simulink library "pbbs_new"  (Simulink 8.1)
settings: Solver=ode1  StartTime=0.0  StopTime=Inf  FixedStep=0.001  RelTol=1e-3
PostLoadFcn:
  | , if any(exist('dsrtsu_mdlpostloadfcn', 'file') == [2, 3, 6]), try dsrtsu_mdlpostloadfcn('Execute', bdroot); catch fprintf('Error in PostLoadFcn (dsrtsu_mdlpostloadfcn) for model "%s":\n %s\n', bdroot, lasterr); end, end,
undefined symbols (not defined in the file or in its folder): KJUD_DecelTGapBraking_s, KJUD_SDFDelay_s, ZERO_FLOAT
libraries: ebdc x1, frdc x1, tbdc x1
settings Model: DSRTSU_INTERNAL_RTI_VER=450  DSRTSU_INTERNAL_RTI_TYPE=rti1401  RTICANMMDATA=struct('GeneralSetupData',struct('modelroot','D:\ELN150201_TAIWAN\trunk\AdasDragon\software\sw_development\arch\app\jud','generalsettings',struct('filesettings',struct('destfolder',struct('Name','RTICANMM_FILES','Check',1),'buildfolder',struct('Name','.','Check',1),'AbsDestfolder',struct('Name','D:\ELN150201_TAIWAN\trunk\AdasDragon\software\sw_development\arch\app\jud\RTICANMM_FILES'),'AbsBuildfolder',struct('Name','D:\ELN150201_TAIWAN\trunk\AdasDragon\software\sw_development\arch\app\jud'))),'options',struct('addpaths',1,'rmpaths',1,'addtrcexclusion',logical(1),'cannavigator',struct('checkmonitoring',0),'show_usrtrc',0,'use_usrtrc',0),'advanced',struct('options',[1 1 1 1 1 1 1 1 1 1 1 1 1 1 1 1 1 1 1 1 1 1 1 1 1 1 1 1 1 1 1 1 1 1 1 1 1 1 1 1 1 1 1 1 1 1 1 1 1 1 1 1 1 1 1 1 1 1 1 1 1 1 1 1 1 1 1 1 1 1 1 1 1 1 1 1 1 1 1 1 1 1 1 1 1 1 1 1 1 1 1 1 1 1 1 1 1 1 1 1]),'MPSetup',{{}},'modelname','pbbs_new','block','pbbs_new'))  DSRTSU_INTERNAL_RTIFPGA=40  Creator=tescamilla  LastModifiedBy=AT015555

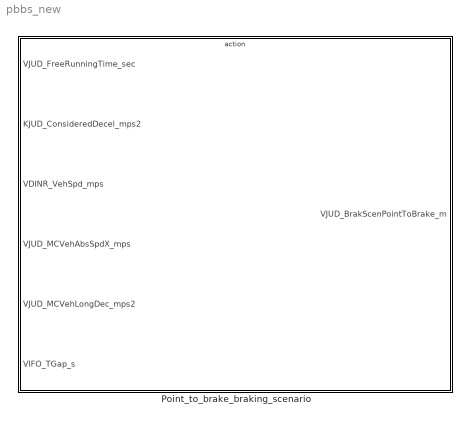
== system pbbs_new ==
  Point_to_brake_braking_scenario : Subsystem

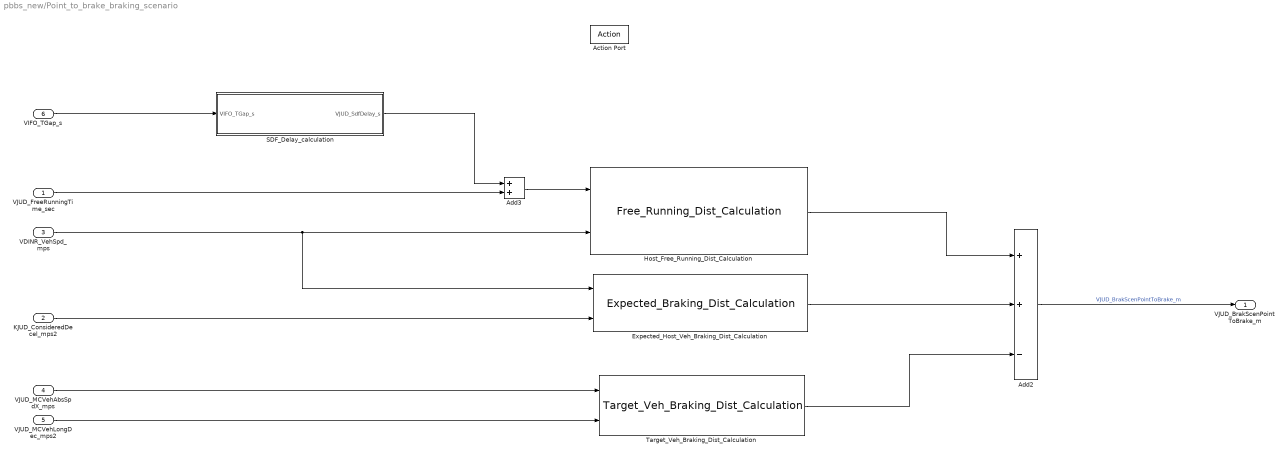
== system pbbs_new/Point_to_brake_braking_scenario ==
  VJUD_FreeRunningTime_sec : Inport
  KJUD_ConsideredDecel_mps2 : Inport  Port=2
  VDINR_VehSpd_mps : Inport  Port=3
  VJUD_MCVehAbsSpdX_mps : Inport  Port=4
  VJUD_MCVehLongDec_mps2 : Inport  Port=5
  VIFO_TGap_s : Inport  Port=6
  Action Port : ActionPort
  Add2 : Sum  Inputs=++-
  Add3 : Sum
  Expected_Host_Veh_Braking_Dist_Calculation : ebdc/Expected_Braking_Dist_Calculation
  Host_Free_Running_Dist_Calculation : frdc/Free_Running_Dist_Calculation
  SDF_Delay_calculation : Subsystem
  Target_Veh_Braking_Dist_Calculation : tbdc/Target_Veh_Braking_Dist_Calculation
  VJUD_BrakScenPointToBrake_m : Outport
  wires:
  KJUD_ConsideredDecel_mps2/1 -> Expected_Host_Veh_Braking_Dist_Calculation/2
  VJUD_FreeRunningTime_sec/1 -> Add3/2
  VDINR_VehSpd_mps/1 -> Expected_Host_Veh_Braking_Dist_Calculation/1, Host_Free_Running_Dist_Calculation/2
  VJUD_MCVehLongDec_mps2/1 -> Target_Veh_Braking_Dist_Calculation/2
  VJUD_MCVehAbsSpdX_mps/1 -> Target_Veh_Braking_Dist_Calculation/1
  Expected_Host_Veh_Braking_Dist_Calculation/1 -> Add2/2
  Host_Free_Running_Dist_Calculation/1 -> Add2/1
  Target_Veh_Braking_Dist_Calculation/1 -> Add2/3
  Add2/1 -> VJUD_BrakScenPointToBrake_m/1  "VJUD_BrakScenPointToBrake_m"
  Add3/1 -> Host_Free_Running_Dist_Calculation/1
  VIFO_TGap_s/1 -> SDF_Delay_calculation/1(VIFO_TGap_s)
  SDF_Delay_calculation/1(VJUD_SdfDelay_s) -> Add3/1

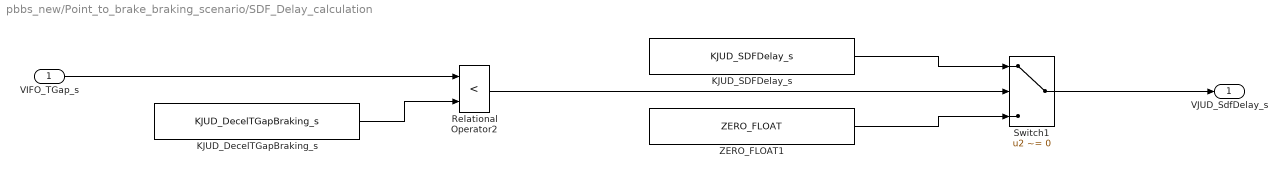
== system pbbs_new/Point_to_brake_braking_scenario/SDF_Delay_calculation ==
  VIFO_TGap_s : Inport
  KJUD_DecelTGapBraking_s : Constant  Value=KJUD_DecelTGapBraking_s  OutDataTypeStr=single
  KJUD_SDFDelay_s : Constant  Value=KJUD_SDFDelay_s
  Relational Operator2 : RelationalOperator  Operator=<  OutDataTypeStr=boolean
  Switch1 : Switch  Criteria=u2 ~= 0
  ZERO_FLOAT1 : Constant  Value=ZERO_FLOAT  OutDataTypeStr=single
  VJUD_SdfDelay_s : Outport
  wires:
  Switch1/1 -> VJUD_SdfDelay_s/1
  KJUD_SDFDelay_s/1 -> Switch1/1
  ZERO_FLOAT1/1 -> Switch1/3
  VIFO_TGap_s/1 -> Relational Operator2/1
  KJUD_DecelTGapBraking_s/1 -> Relational Operator2/2
  Relational Operator2/1 -> Switch1/2
